simulink model "isla_model"  (R2018a)
settings: Solver=VariableStepAuto  StartTime=0.0  StopTime=200  MaxStep=1.3333333333333334E-5  MinStep=1.3333333333333334E-5  RelTol=1e-3
StopFcn:
  | Excitation_Codes;
  | Gap_Code;
undefined symbols (not defined in the file or in its folder): barker, upsample
libraries: dspstat3 x6, dspsrcs4 x5, dspsigops x4, commseqgen3 x2, dspxfrm3 x2, commrflib2 x1
settings Model: Creator=hp  LastModifiedBy=hp
settings SolverCC: InitialStep=1.3333333333333334E-5

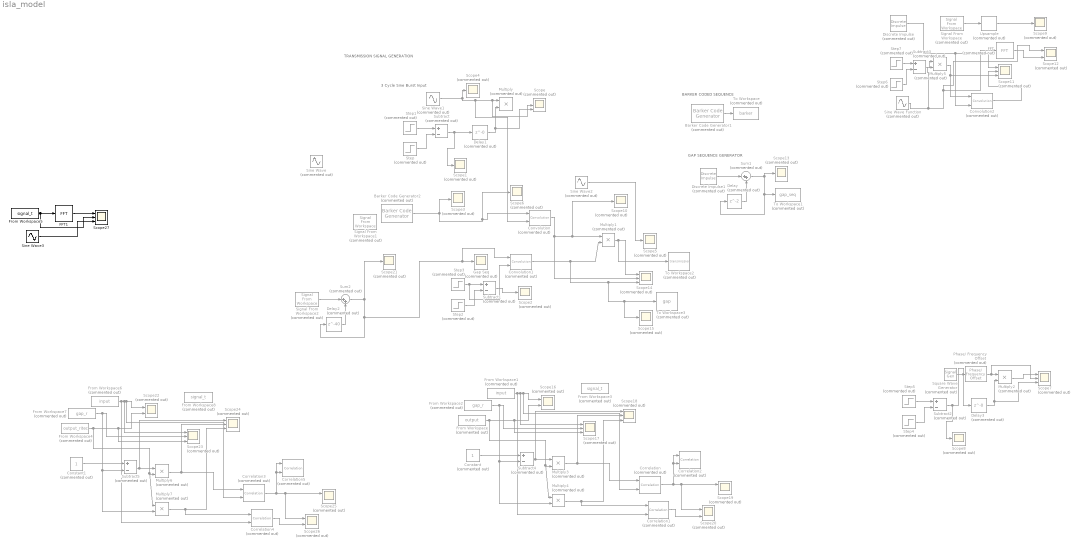
== system isla_model ==
  note: TRANSMISSION SIGNAL GENERATION
  note: BARKER CODED SEQUENCE
  note: 3 Cycle Sine Burst Input
  note: GAP SEQUENCE GENERATOR
  Barker Code Generator1 : commseqgen3/Barker Code Generator  Commented=on  Length=7  LengthSimulink=7  SampleTime=1  SamplesPerFrame=1  OutputDataType=double  SimulateUsing=Code generation
      settings: SourceProductName=Communications System Toolbox  SourceProductBaseCode=CM
  Barker Code Generator2 : commseqgen3/Barker Code Generator  Commented=on  Length=7  LengthSimulink=7  SampleTime=1  SamplesPerFrame=1  OutputDataType=double  SimulateUsing=Code generation
      settings: SourceProductName=Communications System Toolbox  SourceProductBaseCode=CM
  Constant : Constant  Commented=on
  Constant1 : Constant  Commented=on
  Convolution : dspsigops/Convolution  Commented=on  domain=Time  roundingMode=Floor  overflowMode=off  outputDataTypeStr=Inherit: Same as accumulator  outputMin=[]  outputMax=[]  outputLastDataTypeStr=Inherit: Same as accumulator
      settings: SourceProductName=DSP System Toolbox  SourceProductBaseCode=DS
  Convolution1 : dspsigops/Convolution  Commented=on  domain=Time  roundingMode=Floor  overflowMode=off  outputDataTypeStr=Inherit: Same as accumulator  outputMin=[]  outputMax=[]  outputLastDataTypeStr=Inherit: Same as accumulator
      settings: SourceProductName=DSP System Toolbox  SourceProductBaseCode=DS
  Convolution2 : dspsigops/Convolution  Commented=on  domain=Time  roundingMode=Floor  overflowMode=off  accumDataTypeStr=Inherit: Same as product output  accumLastDataTypeStr=Inherit: Same as product output  outputDataTypeStr=Inherit: Same as accumulator  outputMin=[]  outputMax=[]  outputLastDataTypeStr=Inherit: Same as accumulator
      settings: SourceProductName=DSP System Toolbox  SourceProductBaseCode=DS
  Correlation{,1..5} (6 alike) : dspstat3/Correlation  Commented=on  domain=Time  roundingMode=Floor  overflowMode=off  outputDataTypeStr=Inherit: Same as accumulator  outputMin=[]  outputMax=[]  outputLastDataTypeStr=Inherit: Same as accumulator
      settings: SourceProductName=DSP System Toolbox  SourceProductBaseCode=DS
  Delay : Delay  Commented=on
  Delay1 : Delay  Commented=on  DelayLength=0
  Delay2 : Delay  Commented=on  DelayLength=40
  Delay3 : Delay  Commented=on  DelayLength=0
  Discrete Impulse : dspsrcs4/Discrete  Impulse  Commented=on  Delay=[1,2,3,4,5,6,7,8,9,31,32,33,34,35,36,37,38,39]  SampleTime=1  FrameSample=1  OutputFrames=off  dataType=double  isSigned=on  wordLen=16  udDataType=sfix(16)  fracBitsMode=Best precision  numFracBits=15  OutDataTypeStr=double  LastOutDataTypeStr=double
  Discrete Impulse1 : dspsrcs4/Discrete  Impulse  Commented=on  Delay=0  SampleTime=1  FrameSample=1  OutputFrames=off  dataType=double  isSigned=on  wordLen=16  udDataType=sfix(16)  fracBitsMode=Best precision  numFracBits=15  OutDataTypeStr=double  LastOutDataTypeStr=double
  FFT : dspxfrm3/FFT  Commented=on  FFTImplementation=Auto  CompMethod=Table lookup  TableOpt=NEW  TableOptActive=Speed  BitRevOrder=off  Normalize=off  InheritFFTLength=on  FFTLength=64  WrapInput=on  roundingMode=Floor  overflowMode=off  firstCoeffDataTypeStr=Inherit: Same word length as input  firstCoeffLastDataTypeStr=Inherit: Same word length as input  outputMin=[]  outputMax=[]
  FFT1 : dspxfrm3/FFT  FFTImplementation=Auto  CompMethod=Table lookup  TableOpt=NEW  TableOptActive=Speed  BitRevOrder=off  Normalize=off  InheritFFTLength=on  FFTLength=64  WrapInput=on  roundingMode=Floor  overflowMode=off  firstCoeffDataTypeStr=Inherit: Same word length as input  firstCoeffLastDataTypeStr=Inherit: Same word length as input  outputMin=[]  outputMax=[]
  From Workspace : FromWorkspace  Commented=on  VariableName=output  SampleTime=0
  From Workspace1 : FromWorkspace  Commented=on  VariableName=input  SampleTime=0
  From Workspace2 : FromWorkspace  Commented=on  VariableName=gap_r  SampleTime=0
  From Workspace3 : FromWorkspace  Commented=on  VariableName=signal_t  SampleTime=0
  From Workspace4 : FromWorkspace  Commented=on  VariableName=output_ritec  SampleTime=0
  From Workspace5 : FromWorkspace  VariableName=signal_t  SampleTime=0
  From Workspace6 : FromWorkspace  Commented=on  VariableName=input  SampleTime=0
  From Workspace7 : FromWorkspace  Commented=on  VariableName=gap_r  SampleTime=0
  From Workspace8 : FromWorkspace  Commented=on  VariableName=signal_t  SampleTime=0
  "Gap Seq " : Scope  Commented=on
  Multiply{,1..7} (8 alike) : Product  Commented=on
  Phase/ Frequency Offset : commrflib2/Phase// Frequency Offset  Commented=on  phaseOffset=180  freqPort=off  freqOffset=0
      settings: SourceProductName=Communications System Toolbox
  Scope{,7,11,14,17..18,23..24} (8 alike) : Scope  Commented=on  NumInputPorts=3
  Scope{1..6,8..10,13,15,21} (12 alike) : Scope  Commented=on
  Scope{12,16,19..20,22,25..26} (7 alike) : Scope  Commented=on  NumInputPorts=2
  Scope27 : Scope  NumInputPorts=3
  Signal From Workspace : dspsrcs4/Signal From Workspace  Commented=on  X=barker  Ts=1  nsamps=1  OutputAfterFinalValue=Setting to zero  ignoreOrWarnInputAndFrameLengths=off  OutputFrames=off
  Signal From Workspace1 : dspsrcs4/Signal From Workspace  Commented=on  X=upsample(barker, 1)  Ts=1  nsamps=1  OutputAfterFinalValue=Setting to zero  ignoreOrWarnInputAndFrameLengths=off  OutputFrames=off
  Signal From Workspace2 : dspsrcs4/Signal From Workspace  Commented=on  X=gap_seq  Ts=1  nsamps=1  OutputAfterFinalValue=Setting to zero  ignoreOrWarnInputAndFrameLengths=off  OutputFrames=off
  Sine Wave : Sin  Commented=on  Frequency=2*pi  Samples=1000  SampleTime=0.00%.0000001/3
  Sine Wave Function : Sin  Commented=on  SineType=Sample based  Samples=1000  SampleTime=0.001
  Sine Wave1 : Sin  Commented=on  Frequency=2*pi*250000  SampleTime=0
  Sine Wave2 : Sin  Commented=on  Frequency=2*pi*250000  SampleTime=0
  Sine Wave3 : Sin  Frequency=2*pi*250000  SampleTime=0
  Square Wave Generator : SignalGenerator  Commented=on  WaveForm=square  Frequency=0.25
  Step : Step  Commented=on  Time=7%/5*10^4
  Step1 : Step  Commented=on  Time=0
  Step2 : Step  Commented=on  Time=7%/5*10^4  VectorParams1D=off
  Step3 : Step  Commented=on  Time=0  VectorParams1D=off
  Step4 : Step  Commented=on  Time=2
  Step5 : Step  Commented=on  Time=0
  Step6 : Step  Commented=on  Time=5
  Step7 : Step  Commented=on  Time=0
  Subtract{,1..5} (6 alike) : Sum  Commented=on  Inputs=+-
  Sum1 : Sum  Commented=on  Inputs=|++
  Sum2 : Sum  Commented=on  Inputs=|++
  To Workspace : ToWorkspace  Commented=on  VariableName=barker  SampleTime=-1
      settings: Save2DSignal=2-D array (concatenate along first dimension)
  To Workspace1 : ToWorkspace  Commented=on  VariableName=gap_seq  SampleTime=-1
  To Workspace2 : ToWorkspace  Commented=on  VariableName=transmission  SampleTime=-1
      settings: Save2DSignal=2-D array (concatenate along first dimension)
  To Workspace3 : ToWorkspace  Commented=on  VariableName=gap  SampleTime=-1
      settings: Save2DSignal=2-D array (concatenate along first dimension)
  Upsample : dspsigops/Upsample  Commented=on  N=100  phase=0  RateOptions=Allow multirate processing  ic=0  mode=Unused parameter value
  wires:
  Sum1/1 -> To Workspace1/1, Delay/1, Scope13/1
  Step1/1 -> Subtract/1
  Step/1 -> Subtract/2
  Subtract/1 -> Delay1/1, Scope1/1
  Delay1/1 -> Scope/3, Multiply/2
  Step5/1 -> Subtract2/1
  Step4/1 -> Subtract2/2
  Subtract2/1 -> Delay3/1, Scope8/1
  Delay3/1 -> Scope7/3, Multiply2/2
  Multiply2/1 -> Scope7/1
  Square Wave Generator/1 -> Phase/ Frequency Offset/1
  Phase/ Frequency Offset/1 -> Scope7/2, Multiply2/1
  Step2/1 -> Subtract1/2
  Step3/1 -> Convolution1/2, Subtract1/1
  Subtract1/1 -> Scope2/1
  Convolution/1 -> Scope14/2, Scope10/1, Multiply1/1
  Convolution1/1 -> Scope15/1, To Workspace3/1, Scope14/3, Multiply1/2
  Barker Code Generator1/1 -> To Workspace/1
  Signal From Workspace/1 -> Upsample/1
  Upsample/1 -> Scope9/1
  Barker Code Generator2/1 -> Convolution/1, Scope6/1, Scope3/1
  Convolution2/1 -> Scope11/2
  FFT/1 -> Scope12/2
  Sine Wave1/1 -> Scope4/1, Convolution/2, Scope/2, Multiply/1
  Step7/1 -> Subtract3/1
  Step6/1 -> Subtract3/2
  Sine Wave Function/1 -> Multiply5/2, FFT/1, Scope12/1
  Discrete Impulse/1 -> Convolution2/2, Scope11/1
  Delay/1 -> Sum1/2
  Discrete Impulse1/1 -> Sum1/1
  Sum2/1 -> Convolution1/1, "Gap Seq "/1, Delay2/1, Scope21/1
  Multiply1/1 -> To Workspace2/1, Scope14/1
  From Workspace/1 -> Multiply4/1, Multiply3/2, Scope17/3, Scope16/2
  From Workspace2/1 -> Multiply4/2, Subtract4/2, Scope17/2
  Constant/1 -> Subtract4/1
  Subtract4/1 -> Scope18/1, Multiply3/1
  Multiply3/1 -> Scope18/2, Correlation/1
  Correlation/1 -> Scope20/1, Scope19/1, Correlation2/2, Correlation2/1
  From Workspace1/1 -> Correlation1/2, Scope17/1, Correlation/2, Scope16/1
  Multiply4/1 -> Correlation1/1, Scope18/3
  Correlation1/1 -> Scope20/2
  Subtract3/1 -> Multiply5/1
  Multiply5/1 -> Scope11/3, Convolution2/1
  Delay2/1 -> Sum2/2
  Signal From Workspace2/1 -> Sum2/1
  From Workspace6/1 -> Correlation4/2, Scope23/1, Correlation3/2, Scope22/1
  Correlation3/1 -> Scope26/1, Scope25/1, Correlation5/2, Correlation5/1
  Subtract5/1 -> Scope24/1, Multiply6/1
  Multiply7/1 -> Correlation4/1, Scope24/3
  Correlation4/1 -> Scope26/2
  Multiply6/1 -> Scope24/2, Correlation3/1
  From Workspace4/1 -> Multiply7/1, Multiply6/2, Scope23/3, Scope22/2
  Constant1/1 -> Subtract5/1
  From Workspace7/1 -> Multiply7/2, Subtract5/2, Scope23/2
  Sine Wave2/1 -> Scope5/1
  From Workspace5/1 -> Scope27/2, FFT1/1
  FFT1/1 -> Scope27/1
  Sine Wave3/1 -> Scope27/3
